simulink model "Second_Order_Kinematic_Inversion"  (Simulink 9.2)
settings: Solver=VariableStepAuto  StartTime=0.0  StopTime=4  RelTol=1e-3
undefined symbols (not defined in the file or in its folder): DiscIntNeverNeededParam, q0, q0_dot, Tc
settings Model: Creator=sujay  LastModifiedBy=sujay
settings DataIOCC: LimitDataPoints=off  SaveFormat=Dataset  SignalLoggingSaveFormat=Dataset  ReturnWorkspaceOutputs=on
settings OptimizationCC: LifeSpan=auto
settings DebuggingCC: UnderspecifiedInitializationDetection=Simplified  MergeDetectMultiDrivingBlocksExec=error  FcnCallInpInsideContextMsg=error  StateNameClashWarn=none  SFUnexpectedBacktrackingDiag=error  SFNoUnconditionalDefaultTransitionDiag=error  SFExecutionAtInitializationDiag=warning
settings HardwareCC: ProdBitPerPointer=64  ProdBitPerSizeT=64  ProdBitPerPtrDiffT=64  ProdLargestAtomicFloat=Float  ProdIntDivRoundTo=Zero  ProdEndianess=LittleEndian  ProdWordSize=64  ProdHWDeviceType=Intel->x86-64 (Windows64)
settings ModelReferenceCC: PropagateSignalLabelsOutOfModel=on
settings SFSimCC: SimUseLocalCustomCode=on
settings RTWCC: RTWUseLocalCustomCode=on
settings CodeAppCC: StateflowObjectComments=off
settings GRTTargetCC: TargetLangStandard=C99 (ISO)  GeneratePreprocessorConditionals=Use local settings  CombineOutputUpdateFcns=on  GRTInterface=off
settings ConfigComp: CovMetricSettings=dwe  CovHtmlReporting=off  CovSaveCumulativeToWorkspaceVar=off  CovSaveSingleToWorkspaceVar=off  CovExternalEMLEnable=on

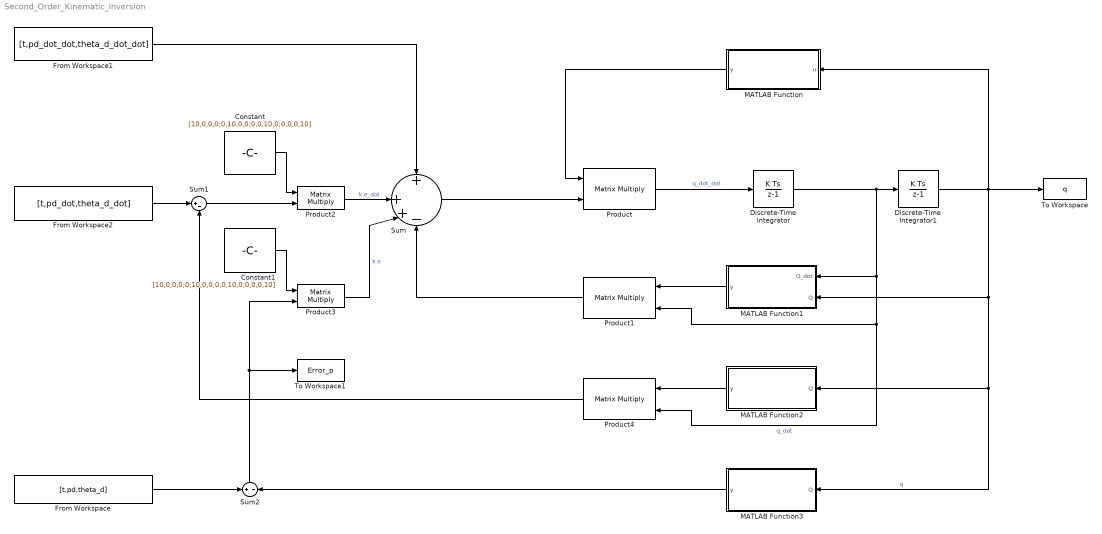
== system Second_Order_Kinematic_Inversion ==
  Constant : Constant  Value=[10,0,0,0;0,10,0,0;0,0,10,0;0,0,0,10]  VectorParams1D=off
  Constant1 : Constant  Value=[10,0,0,0;0,10,0,0;0,0,10,0;0,0,0,10]  VectorParams1D=off
  Discrete-Time Integrator : DiscreteIntegrator  InitialCondition=q0_dot  SampleTime=Tc  ICPrevOutput=DiscIntNeverNeededParam  ICPrevScaledInput=DiscIntNeverNeededParam
  Discrete-Time Integrator1 : DiscreteIntegrator  InitialCondition=q0  SampleTime=Tc  ICPrevOutput=DiscIntNeverNeededParam  ICPrevScaledInput=DiscIntNeverNeededParam
  From Workspace : FromWorkspace  VariableName=[t,pd,theta_d]  SampleTime=0
  From Workspace1 : FromWorkspace  VariableName=[t,pd_dot_dot,theta_d_dot_dot]  SampleTime=0
  From Workspace2 : FromWorkspace  VariableName=[t,pd_dot,theta_d_dot]  SampleTime=0
  MATLAB Function : MATLAB Function  TreatAsAtomicUnit=on
  MATLAB Function1 : MATLAB Function  TreatAsAtomicUnit=on
  MATLAB Function2 : MATLAB Function  TreatAsAtomicUnit=on
  MATLAB Function3 : MATLAB Function  TreatAsAtomicUnit=on
  Product{,1..4} (5 alike) : Product  Multiplication=Matrix(*)
  Sum : Sum  Inputs=+|++-
  Sum1 : Sum  Inputs=|+-
  Sum2 : Sum  Inputs=+|-
  To Workspace : ToWorkspace  VariableName=q  SampleTime=-1
  To Workspace1 : ToWorkspace  VariableName=Error_p  SampleTime=-1
  wires:
  From Workspace/1 -> Sum2/1
  From Workspace1/1 -> Sum/1
  Sum/1 -> Product/2
  MATLAB Function/1(y) -> Product/1
  Product/1 -> Discrete-Time Integrator/1  "q_dot_dot"
  Discrete-Time Integrator/1 -> Product1/2, Product4/2, MATLAB Function1/1(Q_dot), Discrete-Time Integrator1/1  "q_dot"
  Discrete-Time Integrator1/1 -> MATLAB Function2/1(Q), MATLAB Function3/1(Q), MATLAB Function1/2(Q), To Workspace/1, MATLAB Function/1(u)  "q"
  Product1/1 -> Sum/4
  Product2/1 -> Sum/2  "k.e_dot"
  Sum1/1 -> Product2/2
  From Workspace2/1 -> Sum1/1
  Product3/1 -> Sum/3  "k.e"
  Constant/1 -> Product2/1
  Constant1/1 -> Product3/1
  MATLAB Function3/1(y) -> Sum2/2
  Sum2/1 -> To Workspace1/1, Product3/2
  MATLAB Function1/1(y) -> Product1/1
  Product4/1 -> Sum1/2
  MATLAB Function2/1(y) -> Product4/1

== matlab function MATLAB Function1 ==
  data: Q_dot input double; Q input double; y output double
function y = Jacobian_dot(Q_dot,Q)
y = Jacobian_dot(Q,Q_dot);
end

== matlab function MATLAB Function ==
  data: u input double; y output double
function y = Inverse_Jacobian(u)
y = inv(Jacobian(u));
end

== matlab function MATLAB Function2 ==
  data: Q input double; y output double
function y = jacobian(Q)
y = Jacobian(Q);
end

== matlab function MATLAB Function3 ==
  data: Q input double; y output double
function y = Kinematics(Q)
y = [ 0.5*(cos(Q(1,1)+Q(2,1))+cos(Q(1,1))) ; 0.5*(sin(Q(1,1)+Q(2,1))+sin(Q(1,1))) ; (1 - Q(3,1)) ; Q(1,1)+Q(2,1)+Q(4,1) ];
end
